simulink model "veh_driver_model"  (R2017b)
settings: Solver=ode4  StartTime=0.0  StopTime=10  FixedStep=0.001  RelTol=1e-3
values from neighbouring files (symbols this model uses):
  i_sw = 14.5    [Vehicle_Para.m]
  Ts = 0.1    [Vehicle_Para.m]
  Vx_init = 13    [Vehicle_Para.m]
undefined symbols (not defined in the file or in its folder): DiscIntNeverNeededParam, MPC_TO_des_trq, MPC_TO_dri_phase2
libraries: simulink x2
settings Model: Creator=Yutong Li  LastModifiedBy=Yutong Li

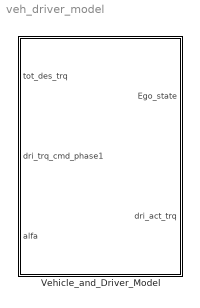
== system veh_driver_model ==
  Vehicle_and_Driver_Model : Subsystem

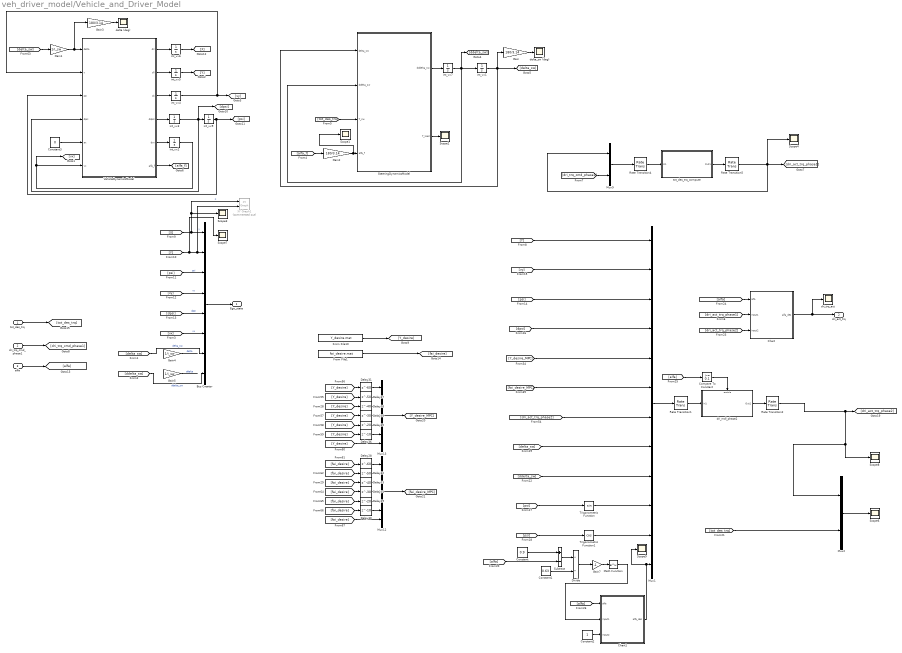
== system veh_driver_model/Vehicle_and_Driver_Model ==
  tot_des_trq : Inport
  dri_trq_cmd_phase1 : Inport  Port=2
  alfa : Inport  Port=3
  Bus Creator : BusCreator  Inputs=8
  Chart : Stateflow chart  TreatAsAtomicUnit=on
  Chart1 : Stateflow chart  TreatAsAtomicUnit=on
  Compare To Constant : simulink/Logic and Bit Operations/Compare To Constant  relop=>=  const=0.1  OutDataTypeStr=boolean
  Constant : Constant  Value=0.9
  Constant1 : Constant  Value=0.63
  Constant2 : Constant
  Constant3 : Constant  Value=0
  Delay28 : Delay  DelayLength=60  InitialCondition=0
  Delay29 : Delay  DelayLength=20  InitialCondition=0
  Delay30 : Delay  DelayLength=10  InitialCondition=0
  Delay31 : Delay  DelayLength=60  InitialCondition=0
  Delay32 : Delay  DelayLength=50  InitialCondition=0
  Delay33 : Delay  DelayLength=40  InitialCondition=0
  Delay34 : Delay  DelayLength=30  InitialCondition=0
  Delay35 : Delay  DelayLength=20  InitialCondition=0
  Delay36 : Delay  DelayLength=10  InitialCondition=0
  Delay37 : Delay  DelayLength=50  InitialCondition=0
  Delay38 : Delay  DelayLength=40  InitialCondition=0
  Delay39 : Delay  DelayLength=30  InitialCondition=0
  Divide : Product  Inputs=*/
  From File1 : FromFile  FileName=fai_desire.mat
  From File10 : FromFile  FileName=Y_desire.mat
  Gain : Gain  Gain=180/3.14
  Gain1 : Gain  Gain=1/i_sw
  Gain2 : Gain  Gain=180/3.14
  Gain3 : Gain  Gain=180/3.14
  Gain4 : Gain  Gain=1/i_sw
  Gain5 : Gain  Gain=1/i_sw
  Gain7 : Gain  Gain=-1
  Math Function : Math  SaturateOnIntegerOverflow=on
  Mux1 : Mux  Inputs=12
  Mux12 : Mux  Inputs=7
  Mux13 : Mux  Inputs=7
  Mux2 : Mux  Inputs=2
  Mux9 : Mux  Inputs=2
  Rate Transition1 : RateTransition  OutPortSampleTime=0.01
  Rate Transition2 : RateTransition
  Rate Transition4 : RateTransition  OutPortSampleTime=0.01
  Rate Transition5 : RateTransition
  Scope{1..4,6..9} (8 alike) : Scope
  SteeringDynamicsModel : MATLAB Function  TreatAsAtomicUnit=on
  Subtract : Sum  Inputs=+-
  Trigonometric Function : Trigonometry
  Trigonometric Function1 : Trigonometry  Operator=cos
  VehicleDynamicsModel : MATLAB Function  TreatAsAtomicUnit=on
  XY Graph1 : simulink/Sinks/XY Graph  Commented=on  xmin=-50  xmax=300  ymin=-5  ymax=70  st=-1
  delta (deg) : Scope
  delta_sw (deg) : Scope
  dri_mdl_phase2 : Subsystem  TreatAsAtomicUnit=on
  dri_trq_act : Scope
  int_vx1 : Integrator  LimitOutput=on  UpperSaturationLimit=360/180*3.14  LowerSaturationLimit=-360/180*3.14
  int_vx2 : Integrator  InitialCondition=Vx_init
  int_vx{3..7,9} (6 alike) : Integrator
  tot_des_trq_compute : Subsystem  TreatAsAtomicUnit=on
  Ego_state : Outport
  dri_act_trq : Outport  Port=2
  wires:
  [Y] -> Scope7/1, XY Graph1/2, Bus Creator/2  "Y"
  [psi] -> Bus Creator/3  "psi"
  Bus Creator/1 -> Ego_state/1
  [vy] -> Bus Creator/4  "vy"
  [dpsi] -> Bus Creator/5  "dpsi"
  [X] -> XY Graph1/1, Scope3/1, Bus Creator/1  "X"
  [vx] -> Bus Creator/6  "vx"
  VehicleDynamicsModel/2(dY) -> int_vx5/1
  VehicleDynamicsModel/3(dv) -> int_vx4/1
  int_vx4/1 -> VehicleDynamicsModel/2(v), [vy]
  int_vx6/1 -> [X]
  VehicleDynamicsModel/1(dX) -> int_vx6/1
  int_vx5/1 -> [Y]
  VehicleDynamicsModel/4(ddpsi) -> int_vx3/1
  int_vx3/1 -> [dpsi], int_vx9/1, VehicleDynamicsModel/4(dpsi)
  int_vx9/1 -> [psi], VehicleDynamicsModel/3(psi)
  Constant3/1 -> VehicleDynamicsModel/5(ax)
  VehicleDynamicsModel/5(dvx) -> int_vx2/1
  int_vx2/1 -> [vx], VehicleDynamicsModel/6(vx)
  tot_des_trq/1 -> [tot_des_trq]
  [delta_sw] -> Gain1/1
  int_vx7/1 -> [ddelta_sw], SteeringDynamicsModel/2(ddelta_sw), int_vx1/1
  SteeringDynamicsModel/1(dddelta_sw) -> int_vx7/1
  int_vx1/1 -> Gain/1, [delta_sw], SteeringDynamicsModel/1(delta_sw)
  [delta_sw] -> Bus Creator/7  "delta_sw"
  [ddelta_sw] -> Bus Creator/8  "ddelta_sw"
  [tot_des_trq] -> SteeringDynamicsModel/3(T_sw)
  SteeringDynamicsModel/2(T_load) -> Scope2/1
  Gain/1 -> delta_sw (deg)/1
  VehicleDynamicsModel/6(alfa_f) -> [alfa_f]
  [alfa_f] -> Gain2/1
  Gain1/1 -> Gain3/1, VehicleDynamicsModel/1(delta)
  Gain2/1 -> Scope1/1, SteeringDynamicsModel/4(alfa_f)
  Gain3/1 -> delta (deg)/1
  Gain4/1 -> ?  "delta"
  Gain5/1 -> ?  "ddelta"
  [dri_act_trq_phase1] -> Chart/2(input1)
  dri_trq_cmd_phase1/1 -> [dri_trq_cmd_phase1]
  Rate Transition5/1 -> [dri_act_trq_phase1], Scope4/1, Mux9/1
  Mux9/1 -> Rate Transition4/1
  tot_des_trq_compute/1(Out1) -> Rate Transition5/1
  Rate Transition4/1 -> tot_des_trq_compute/1(In1)
  [dri_trq_cmd_phase1] -> Mux9/2
  Trigonometric Function/1 -> Mux1/10
  Trigonometric Function1/1 -> Mux1/11
  [delta_sw] -> Mux1/8
  [psi] -> Trigonometric Function/1
  [fai_desire_MPC] -> Mux1/6
  [Y_desire_MPC] -> Mux1/5
  dri_mdl_phase2/1(Out1) -> Rate Transition2/1
  [psi] -> Trigonometric Function1/1
  [dpsi] -> Mux1/4
  [vy] -> Mux1/2
  [Y] -> Mux1/1
  Rate Transition1/1 -> dri_mdl_phase2/1(In1)
  Mux1/1 -> Rate Transition1/1
  [ddelta_sw] -> Mux1/9
  [dri_act_trq_phase2] -> Mux1/7
  [psi] -> Mux1/3
  From File10/1 -> [Y_desire]
  From File1/1 -> [fai_desire]
  Delay34/1 -> Mux12/4
  Delay38/1 -> Mux13/3
  Delay37/1 -> Mux13/2
  Delay33/1 -> Mux12/3
  Delay36/1 -> Mux13/6
  [fai_desire] -> Delay33/1
  Delay32/1 -> Mux12/2
  [fai_desire] -> Delay29/1
  Mux12/1 -> [fai_desire_MPC]
  [Y_desire] -> Delay37/1
  [Y_desire] -> Delay31/1
  Mux13/1 -> [Y_desire_MPC]
  [Y_desire] -> Delay38/1
  Delay29/1 -> Mux12/5
  [Y_desire] -> Delay39/1
  Delay30/1 -> Mux12/6
  [Y_desire] -> Delay36/1
  [Y_desire] -> Mux13/7
  Delay28/1 -> Mux12/1
  [fai_desire] -> Delay30/1
  [fai_desire] -> Delay34/1
  Delay35/1 -> Mux13/5
  [fai_desire] -> Delay32/1
  Delay31/1 -> Mux13/1
  Delay39/1 -> Mux13/4
  [fai_desire] -> Delay28/1
  [fai_desire] -> Mux12/7
  [Y_desire] -> Delay35/1
  alfa/1 -> [alfa]
  [tot_des_trq] -> Mux2/2
  Mux2/1 -> Scope6/1
  Constant/1 -> Subtract/1
  Subtract/1 -> Divide/1
  Divide/1 -> Gain7/1
  Gain7/1 -> Math Function/1
  [dri_act_trq_phase2] -> Chart/3(input2)
  [alfa] -> Chart/1(alfa)
  Chart/1(alfa_des) -> dri_trq_act/1, dri_act_trq/1
  [alfa] -> Compare To Constant/1
  Compare To Constant/1 -> dri_mdl_phase2/Enable
  Rate Transition2/1 -> Scope8/1, Mux2/1, [dri_act_trq_phase2]
  [alfa] -> Subtract/2
  Math Function/1 -> Chart1/2(input1)
  Chart1/1(alfa_des) -> Scope9/1, Mux1/12
  [alfa] -> Chart1/1(alfa)
  Constant2/1 -> Chart1/3(input2)
  Constant1/1 -> Divide/2

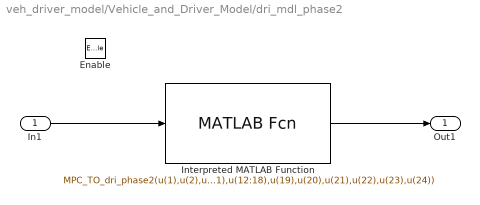
== system veh_driver_model/Vehicle_and_Driver_Model/dri_mdl_phase2 ==
  In1 : Inport
  Enable : EnablePort
  Interpreted MATLAB Function : MATLABFcn  MATLABFcn=MPC_TO_dri_phase2(u(1),u(2),u(3),u(4),u(5:11),u(12:18),u(19),u(20),u(21),u(22),u(23),u(24))  OutputDimensions=1  SampleTime=0.01
  Out1 : Outport
  wires:
  In1/1 -> Interpreted MATLAB Function/1
  Interpreted MATLAB Function/1 -> Out1/1

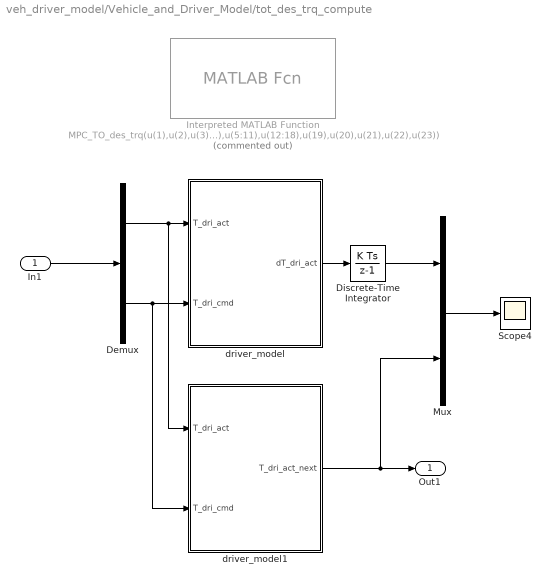
== system veh_driver_model/Vehicle_and_Driver_Model/tot_des_trq_compute ==
  In1 : Inport
  Demux : Demux  Outputs=2
  Discrete-Time Integrator : DiscreteIntegrator  InitialConditionSetting=State (most efficient)  SampleTime=Ts  ICPrevOutput=DiscIntNeverNeededParam  ICPrevScaledInput=DiscIntNeverNeededParam
  Interpreted MATLAB Function : MATLABFcn  Commented=on  MATLABFcn=MPC_TO_des_trq(u(1),u(2),u(3),u(4),u(5:11),u(12:18),u(19),u(20),u(21),u(22),u(23))  OutputDimensions=1  SampleTime=Ts
  Mux : Mux  Inputs=2
  Scope4 : Scope
  driver_model : MATLAB Function  TreatAsAtomicUnit=on
  driver_model1 : MATLAB Function  TreatAsAtomicUnit=on
  Out1 : Outport
  wires:
  In1/1 -> Demux/1
  driver_model/1(dT_dri_act) -> Discrete-Time Integrator/1
  Demux/1 -> driver_model1/1(T_dri_act), driver_model/1(T_dri_act)
  Demux/2 -> driver_model1/2(T_dri_cmd), driver_model/2(T_dri_cmd)
  driver_model1/1(T_dri_act_next) -> Mux/2, Out1/1
  Discrete-Time Integrator/1 -> Mux/1
  Mux/1 -> Scope4/1

== matlab function veh_driver_model/Vehicle_and_Driver_Model/VehicleDynamicsModel ==
  data: dX output; delta input; dY output; v input; dv output; psi input; dpsi input; ddpsi output; ax input; dvx output; vx input; alfa_f output
function [dX,dY, dv, ddpsi, dvx, alfa_f] = fcn(delta, v, psi, dpsi, ax, vx)
% persistent K_f K_r b_f b_r alfa_f alfa_r
m = 1830;
lf = 1.152;
lr = 1.693;
Iz = 3477;


K_f = 40703*2;
K_r = 64495*2;


alfa_f = (v + dpsi*lf)/vx - delta;
alfa_r = (v - dpsi*lr)/vx;
Fy_f = -K_f*alfa_f;
Fy_r = -K_r*alfa_r;

dvx = ax;
dv = -vx*dpsi + 1/m*(Fy_f + Fy_r);
ddpsi = 1/Iz*(lf*Fy_f - lr*Fy_r);
dX = vx*cos(psi) - v*sin(psi);
dY = vx*sin(psi) + v*cos(psi);

== matlab function veh_driver_model/Vehicle_and_Driver_Model/SteeringDynamicsModel ==
  data: dddelta_sw output; delta_sw input; ddelta_sw input; T_sw input; T_load output; alfa_f input
function [dddelta_sw, T_load]  = fcn(delta_sw, ddelta_sw, T_sw, alfa_f)
% persistent K_f K_r b_f b_r alfa_f alfa_r

K_sw = 2.29*6;
B_sw = 1.56/2;
J_sw = 0.172;
is = 14.5;
K_load = 30;
K_sw_load = K_load*0.4;


T_load = -K_sw_load*alfa_f/is;
dddelta_sw = -K_sw/J_sw*delta_sw - B_sw/J_sw*ddelta_sw + 1/J_sw*(T_sw - T_load);

== matlab function veh_driver_model/Vehicle_and_Driver_Model/tot_des_trq_compute/driver_model ==
  data: T_dri_act input; T_dri_cmd input; dT_dri_act output
function dT_dri_act  = fcn( T_dri_act, T_dri_cmd)
% persistent K_f K_r b_f b_r alfa_f alfa_r

tao_driver = 0.5;

K = 7; 

dT_dri_act = -1/tao_driver*T_dri_act + K/tao_driver*T_dri_cmd;

== matlab function veh_driver_model/Vehicle_and_Driver_Model/tot_des_trq_compute/driver_model1 ==
  data: T_dri_act input; T_dri_cmd input; T_dri_act_next output
function T_dri_act_next  = fcn( T_dri_act, T_dri_cmd)
% persistent K_f K_r b_f b_r alfa_f alfa_r

tao_driver = .5;

K = 7; 

T_s = 0.01;

T_dri_act_next = (1 - T_s/tao_driver)*T_dri_act + K*T_s/tao_driver*T_dri_cmd;

== stateflow chart veh_driver_model/Vehicle_and_Driver_Model/Chart ==
  state state_1
    during:
    alfa_des = input1;
  state state_2
    during:
    alfa_des = input2;
  (default) -> state_1
  state_1 -> state_2 : [alfa>0.6]
  data: alfa input; input1 input; alfa_des output; input2 input

== stateflow chart veh_driver_model/Vehicle_and_Driver_Model/Chart1 ==
  state state_1
    during:
    alfa_des = input1;
  state state_2
    during:
    alfa_des = 1;
  (default) -> state_1
  state_1 -> state_2 : [alfa>0.9]
  data: alfa input; input1 input; alfa_des output; input2 input
